simulink model "w3_prob2_214869"  (R2020a)
settings: Solver=FixedStepDiscrete  StartTime=0.0  StopTime=150  FixedStep=.1  RelTol=1e-3  EnableMultiTasking=on
undefined symbols (not defined in the file): DiscIntNeverNeededParam
libraries: simulink x1
settings Model: DataDictionary=w3_prob2.sldd  Creator=sonal  LastModifiedBy=sonal
settings DataIOCC: LimitDataPoints=on  SaveFormat=Array

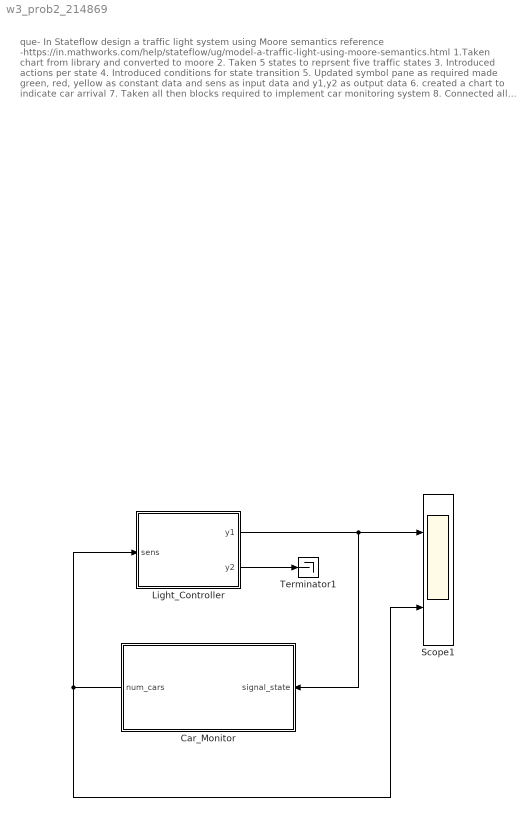
== system w3_prob2_214869 ==
  note: que- In Stateflow design a traffic light system using Moore semantics
      | reference -https://in.mathworks.com/help/stateflow/ug/model-a-traffic-light-using-moore-semantics.html
      |
      | 1.Taken chart from library and converted to moore
      | 2. Taken 5 states to reprsent five traffic states
      | 3. Introduced actions per state
      | 4. Introduced conditions for state transition
      | 5. Updated symbol pane as required
      | made green, red, yellow as constant data and sens as input data and y1,y2 as output data
      | 6. created a chart to indicate car arrival
      | 7. Taken all then blocks required to implement car monitoring system
      | 8. Connected all the blocks to model traffic
      | 9. Created a subsystem from all the blocks and given name car_monitor
      | 10. Created data dictionary for parameters
      | 11. Selected stop time=150 and solver= fixed step discrete
      | 12. updated value of red, green, yellow as 1,2,3 respectively in symbol pane
  Car_Monitor : Subsystem
  Light_Controller : Stateflow chart  TreatAsAtomicUnit=on
  Scope1 : Scope  NumInputPorts=2
  Terminator1 : Terminator
  wires:
  Car_Monitor/1(num_cars) -> Scope1/2, Light_Controller/1(sens)
  Light_Controller/1(y1) -> Scope1/1, Car_Monitor/1(signal_state)
  Light_Controller/2(y2) -> Terminator1/1

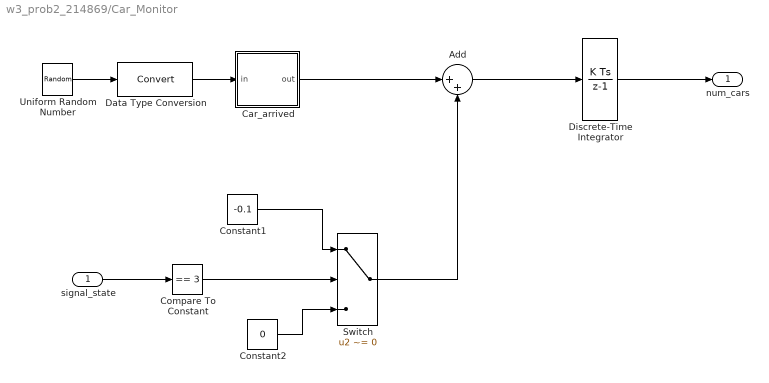
== system w3_prob2_214869/Car_Monitor ==
  signal_state : Inport
  Add : Sum  Inputs=|++
  Car_arrived : Stateflow chart  TreatAsAtomicUnit=on
  Compare To Constant : simulink/Logic and Bit Operations/Compare To Constant  relop===  const=3  OutDataTypeStr=boolean  ZeroCross=off
  Constant1 : Constant  Value=-0.1
  Constant2 : Constant  Value=0
  Data Type Conversion : DataTypeConversion
  Discrete-Time Integrator : DiscreteIntegrator  SampleTime=-1  LimitOutput=on  LowerSaturationLimit=0  ICPrevOutput=DiscIntNeverNeededParam  ICPrevScaledInput=DiscIntNeverNeededParam
  Switch : Switch  Criteria=u2 ~= 0
  Uniform Random Number : UniformRandomNumber  Minimum=0  Maximum=100  Seed=177836  SampleTime=0
  num_cars : Outport  VectorParamsAs1DForOutWhenUnconnected=off
  wires:
  Constant1/1 -> Switch/1
  Constant2/1 -> Switch/3
  Discrete-Time Integrator/1 -> num_cars/1
  signal_state/1 -> Compare To Constant/1
  Compare To Constant/1 -> Switch/2
  Switch/1 -> Add/2
  Add/1 -> Discrete-Time Integrator/1
  Car_arrived/1(out) -> Add/1
  Data Type Conversion/1 -> Car_arrived/1(in)
  Uniform Random Number/1 -> Data Type Conversion/1

== stateflow chart w3_prob2_214869/Light_Controller ==
  settings: stateMachineType=MOORE_MACHINE  executeAtInitialization=1  initializeOutput=1
  state Stop
    y1 = red;
    y2 = green;
  state stop_for_traffic
    y1 = red;
    y2 = green;
  state stop_to_Go
    y1 = red;
    y2 = yellow;
  state Go_to_stop
    y1 = yellow;
    y2 = red;
  state Go
    y1 = green;
    y2 = red;
  (default) -> Stop
  stop_for_traffic -> stop_to_Go : [sens]
  Stop -> stop_for_traffic : after(20,tick)
  Go_to_stop -> Stop : after (3,tick)
  stop_to_Go -> Go : after(3,tick)
  Go -> Go_to_stop : after(10,tick)
  data: sens input double; y1 output double; y2 output double; green constant double =3; yellow constant double =2; red constant double =1

== stateflow chart w3_prob2_214869/Car_Monitor/Car_arrived ==
  (default) -> (junction 2) : {out = in > 98;}
  data: in input int8; out output double
